simulink model "Abs6"  (Simulink 9.0)
settings: Solver=FixedStepDiscrete  StartTime=0.0  StopTime=10.0  FixedStep=1.000000  RelTol=1e-3  EnableMultiTasking=on
settings Model: SuppressorTable=22 serialization::archive 11 0 6 0 0 0 0 0  Creator=arnaud  LastModifiedBy=hbourbou
settings DataIOCC: LimitDataPoints=on  SaveFormat=Structure  SignalLoggingSaveFormat=ModelDataLogs
settings OptimizationCC: ExpressionDepthLimit=2147483647
settings DebuggingCC: SolverPrmCheckMsg=warning  FcnCallInpInsideContextMsg=warning  StateNameClashWarn=warning
settings GRTTargetCC: GeneratePreprocessorConditionals=Disable all  CombineOutputUpdateFcns=off  GRTInterface=on
settings ConfigComp: CovSFcnEnable=off

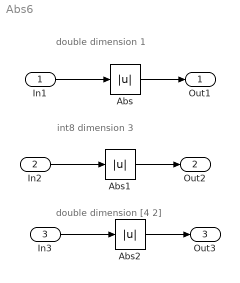
== system Abs6 ==
  note: double dimension [4 2]
  note: int8 dimension 3
  note: double dimension 1
  In1 : Inport  OutDataTypeStr=double
  In2 : Inport  Port=2  OutDataTypeStr=int8  PortDimensions=[3]
  In3 : Inport  Port=3  PortDimensions=[4 2]
  Abs : Abs
  Abs1 : Abs
  Abs2 : Abs
  Out1 : Outport
  Out2 : Outport  Port=2
  Out3 : Outport  Port=3
  wires:
  In1/1 -> Abs/1
  Abs/1 -> Out1/1
  In2/1 -> Abs1/1
  Abs1/1 -> Out2/1
  In3/1 -> Abs2/1
  Abs2/1 -> Out3/1
